simulink model "check_ndtm_variableFriction"  (R2018b)
settings: Solver=FixedStepAuto  StartTime=0.0  StopTime=50  FixedStep=tSPhysics  RelTol=1e-3
settings Model: DataDictionary=check_ndtm.sldd  Creator=staer  LastModifiedBy=staer

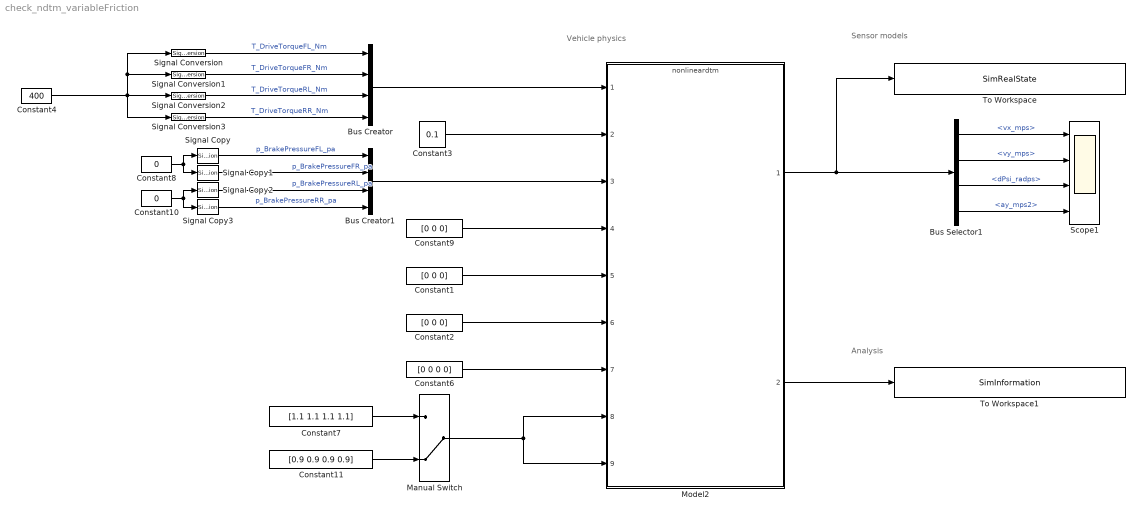
== system check_ndtm_variableFriction ==
  note: Analysis
  note: Vehicle physics
  note: Sensor models
  Bus Creator : BusCreator  Inputs=4  OutDataTypeStr=Bus: DriveTorque_Nm
  Bus Creator1 : BusCreator  Inputs=4  OutDataTypeStr=Bus: BrakePressure_Pa
  Bus Selector1 : BusSelector  OutputSignals=vx_mps,vy_mps,dPsi_radps,ay_mps2
  Constant1 : Constant  Value=[0 0 0]
  Constant10 : Constant  Value=0
  Constant11 : Constant  Value=[0.9 0.9 0.9 0.9]
  Constant2 : Constant  Value=[0 0 0]
  Constant3 : Constant  Value=0.1
  Constant4 : Constant  Value=400
  Constant6 : Constant  Value=[0 0 0 0]
  Constant7 : Constant  Value=[1.1 1.1 1.1 1.1]
  Constant8 : Constant  Value=0
  Constant9 : Constant  Value=[0 0 0]
  Manual Switch : ManualSwitch  CurrentSetting=0
  Model2 : ModelReference  ModelNameDialog=nonlineardtm  ParameterArgumentNames=x0_initialstates  ParameterArgumentValues=[0 0 0 0 0 -pi/2]  UsingDefaultArgumentValue=0  SimulationMode=Normal  ModelReferenceVersion=1.710
  Scope1 : Scope  NumInputPorts=4
  Signal Conversion{,1..3} (4 alike) : SignalConversion  OverrideOpt=off
  Signal Copy{,1..3} (4 alike) : SignalConversion  OverrideOpt=off
  To Workspace : ToWorkspace  VariableName=SimRealState  SaveFormat=Timeseries  SampleTime=-1
  To Workspace1 : ToWorkspace  VariableName=SimInformation  SaveFormat=Timeseries  SampleTime=-1
  wires:
  Signal Copy/1 -> Bus Creator1/1  "p_BrakePressureFL_pa"
  Bus Selector1/1 -> Scope1/1  "<vx_mps>"
  Constant10/1 -> Signal Copy3/1, Signal Copy2/1
  Bus Creator/1 -> Model2/1
  Bus Selector1/4 -> Scope1/4  "<ay_mps2>"
  Bus Selector1/2 -> Scope1/2  "<vy_mps>"
  Signal Copy1/1 -> Bus Creator1/2  "p_BrakePressureFR_pa"
  Signal Copy3/1 -> Bus Creator1/4  "p_BrakePressureRR_pa"
  Signal Conversion2/1 -> Bus Creator/3  "T_DriveTorqueRL_Nm"
  Constant2/1 -> Model2/6
  Signal Conversion3/1 -> Bus Creator/4  "T_DriveTorqueRR_Nm"
  Bus Selector1/3 -> Scope1/3  "<dPsi_radps>"
  Signal Conversion/1 -> Bus Creator/1  "T_DriveTorqueFL_Nm"
  Bus Creator1/1 -> Model2/3
  Signal Conversion1/1 -> Bus Creator/2  "T_DriveTorqueFR_Nm"
  Constant8/1 -> Signal Copy1/1, Signal Copy/1
  Signal Copy2/1 -> Bus Creator1/3  "p_BrakePressureRL_pa"
  Model2/1 -> Bus Selector1/1, To Workspace/1
  Constant6/1 -> Model2/7
  Constant1/1 -> Model2/5
  Constant4/1 -> Signal Conversion/1, Signal Conversion1/1, Signal Conversion3/1, Signal Conversion2/1
  Constant9/1 -> Model2/4
  Manual Switch/1 -> Model2/9, Model2/8
  Model2/2 -> To Workspace1/1
  Constant3/1 -> Model2/2
  Constant7/1 -> Manual Switch/1
  Constant11/1 -> Manual Switch/2
